simulink model "LiepkePlane"  (R2021a)
settings: Solver=FixedStepDiscrete  StartTime=0.0  StopTime=100  RelTol=1e-3  EnableMultiTasking=on
InitFcn:
  | runStart
StopFcn:
  | createGraphs
values from neighbouring files (symbols this model uses):
  alpha_matrix = data.alpha    [DatcomImport.m]
  alphai = trimAngle    (= -0.08927272)    [runStart.m]
  alt_matrix = data.alt    [DatcomImport.m]
  b = 8.0162    [runStart.m]
  beta = 0    [runStart.m]
  cbar = 4.3    [runStart.m]
  CD_0 = 0.0205    [runStart.m]
  CD_alpha = 0.058388    [runStart.m]
  CD_de = 0    [runStart.m]
  CD_ih = 0    [runStart.m]
  CD_q = 0    [runStart.m]
  CL_0 = 0.149    [runStart.m]
  Cl_0 = 0    [runStart.m]
  CL_alpha = 5.1265    [runStart.m]
  Cl_beta = -0.0301    [runStart.m]
  Cl_da = -0.1    [runStart.m]
  CL_de = 0.38    [runStart.m]
  Cl_dr = 0.05    [runStart.m]
  CL_ih = 0    [runStart.m]
  Cl_p = -0.5    [runStart.m]
  CL_q = 10.0    (= 10)    [runStart.m]
  Cl_r = 0.28    [runStart.m]
  cla_matrix = data.cla    [DatcomImport.m]
  clb_matrix = data.clb    [DatcomImport.m]
  clp_matrix = data.clp    [DatcomImport.m]
  clq_matrix = data.clq    [DatcomImport.m]
  clr_matrix = data.clr    [DatcomImport.m]
  Cm_0 = -0.08    [runStart.m]
  Cm_alpha = -0.3109    [runStart.m]
  Cm_de = -0.88    [runStart.m]
  Cm_ih = 0    [runStart.m]
  Cm_q = -17.7    [runStart.m]
  cma_matrix = data.cma    [DatcomImport.m]
  cmq_matrix = data.cmq    [DatcomImport.m]
  Cn_0 = 0    [runStart.m]
  Cn_beta = 0.1297    [runStart.m]
  Cn_da = 0.003    [runStart.m]
  Cn_dr = -0.18436    [runStart.m]
  Cn_p = - 0.09    (= -0.09)    [runStart.m]
  Cn_r = -0.26    [runStart.m]
  cnb_matrix = data.cnb    [DatcomImport.m]
  cnp_matrix = data.cnp    [DatcomImport.m]
  cnr_matrix = data.cnr    [DatcomImport.m]
  CY_0 = 0    [runStart.m]
  CY_beta = -.0301    (= -0.0301)    [runStart.m]
  CY_da = 0    [runStart.m]
  CY_dr = 0.0280    (= 0.028)    [runStart.m]
  CY_p = -0.140    (= -0.14)    [runStart.m]
  CY_r = 0.61    [runStart.m]
  cyb_matrix = data.cyb    [DatcomImport.m]
  cyp_matrix = data.cyp    [DatcomImport.m]
  H = 1981.2    [runStart.m]
  Ix = 1084.7    [runStart.m]
  Iy = 6507.9    [runStart.m]
  Iz = 7050.3    [runStart.m]
  Jxy = 0    [runStart.m]
  Jxz = 271.16    [runStart.m]
  Jyz = 0    [runStart.m]
  m = 2267.9    [runStart.m]
  mach_matrix = data.mach    [DatcomImport.m]
  p = 0    [runStart.m]
  phi = 0    [runStart.m]
  psi = 0    [runStart.m]
  q = 0    [runStart.m]
  r = 0    [runStart.m]
  S = 12.6348    [runStart.m]
  theta = trimAngle    (= -0.08927272)    [runStart.m]
  trimAngle = -8.927272e-02    (= -0.08927272)    [runStart.m]
  trimThrotte = 3.827652e-01    (= 0.3827652)    [runStart.m]
  v = 180    [runStart.m]
  xe = 0    [runStart.m]
  ye = 0    [runStart.m]
undefined symbols (not defined in the file or in its folder): DiscIntNeverNeededParam
libraries: airlib x2, aerolibfltsims x2, aerolibanimutils x2
(part 2 of 2)

== system LiepkePlane/ Liepke - AE 413 FInal/ae/aero/Stability 2 Body Axis ==
  alpha : Inport
  FsMb : Inport  Port=2
  Demux2 : Demux  Outputs=6
      settings: DisplayOption=none
  Mux1 : Mux  Inputs=6
  Product{2..5} (4 alike) : Product  InputSameDT=on  RndMeth=Zero  SaturateOnIntegerOverflow=on  OutDataTypeStr=Inherit: Same as first input
  Sum3 : Sum  Inputs=-+  InputSameDT=on  SaturateOnIntegerOverflow=on  OutDataTypeStr=Inherit: Same as first input
  Sum4 : Sum  Inputs=--  InputSameDT=on  SaturateOnIntegerOverflow=on  OutDataTypeStr=Inherit: Same as first input
  cos alpha : Fcn  Expr=cos(u[1])
  sin alpha : Fcn
  FbMb : Outport  VectorParamsAs1DForOutWhenUnconnected=off
  wires:
  Demux2/6 -> Mux1/6
  Demux2/5 -> Mux1/5
  Demux2/2 -> Mux1/2
  Demux2/4 -> Mux1/4
  cos alpha/1 -> Product2/1, Product5/1
  Demux2/1 -> Product2/2, Product4/2
  Product2/1 -> Sum3/1
  Product3/1 -> Sum3/2
  Sum3/1 -> Mux1/1
  sin alpha/1 -> Product3/1, Product4/1
  Demux2/3 -> Product3/2, Product5/2
  Product4/1 -> Sum4/1
  Product5/1 -> Sum4/2
  Sum4/1 -> Mux1/3
  alpha/1 -> sin alpha/1, cos alpha/1
  Mux1/1 -> FbMb/1
  FsMb/1 -> Demux2/1

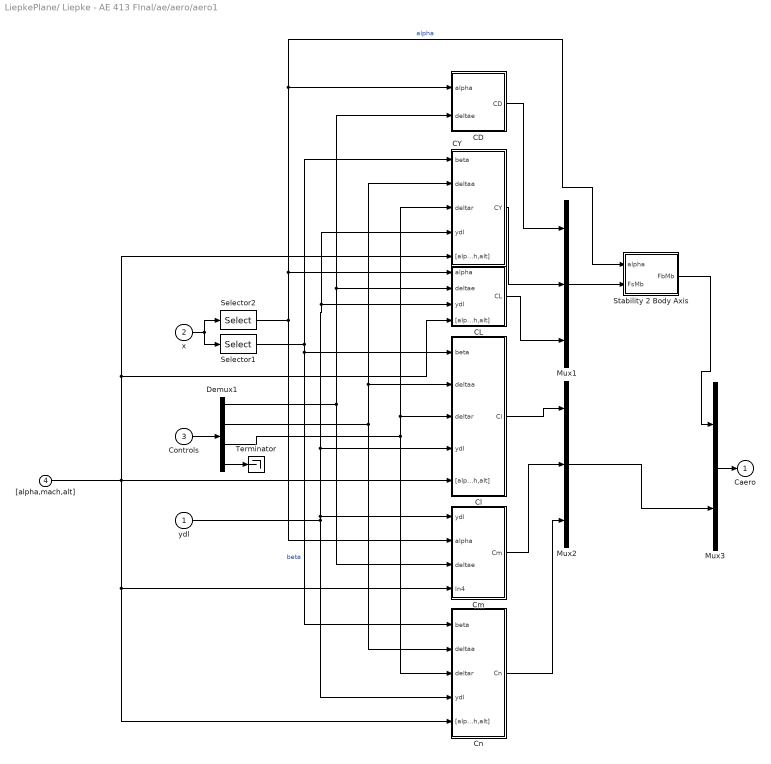
== system LiepkePlane/ Liepke - AE 413 FInal/ae/aero/aero1 ==
  ydl : Inport
  x : Inport  Port=2
  Controls : Inport  Port=3
  "[alpha,mach,alt]" : Inport  Port=4
  CD : Subsystem
  CL : Subsystem
  CY : Subsystem
  Cl : Subsystem
  Cm : Subsystem
  Cn : Subsystem
  Demux1 : Demux
      settings: DisplayOption=none
  Mux1 : Mux  Inputs=3
  Mux2 : Mux  Inputs=3
  Mux3 : Mux  Inputs=2
  Selector1 : Selector  InputPortWidth=12  IndexOptions=Index vector (dialog)  Indices=[3]  OutputSizes=1
  Selector2 : Selector  InputPortWidth=12  IndexOptions=Index vector (dialog)  Indices=[2]  OutputSizes=1
  Stability 2 Body Axis : Subsystem
  Terminator : Terminator
  Caero : Outport  VectorParamsAs1DForOutWhenUnconnected=off
  wires:
  Demux1/3 -> CY/3(deltar), Cl/3(deltar), Cn/3(deltar)
  Demux1/2 -> CY/2(deltaa), Cl/2(deltaa), Cn/2(deltaa)
  Demux1/1 -> CD/2(deltae), CL/2(deltae), Cm/3(deltae)
  ydl/1 -> CY/4(ydl), CL/3(ydl), Cl/4(ydl), Cm/1(ydl), Cn/4(ydl)
  CD/1(CD) -> Mux1/1
  Mux1/1 -> Stability 2 Body Axis/2(FsMb)
  CY/1(CY) -> Mux1/2
  x/1 -> Selector2/1, Selector1/1
  Selector1/1 -> Cn/1(beta), Cl/1(beta), CY/1(beta)  "beta"
  Selector2/1 -> Cm/2(alpha), Stability 2 Body Axis/1(alpha), CD/1(alpha), CL/1(alpha)  "alpha"
  CL/1(CL) -> Mux1/3
  Controls/1 -> Demux1/1
  Demux1/4 -> Terminator/1
  Stability 2 Body Axis/1(FbMb) -> Mux3/1
  Cl/1(Cl) -> Mux2/1
  Cm/1(Cm) -> Mux2/2
  Cn/1(Cn) -> Mux2/3
  Mux3/1 -> Caero/1
  Mux2/1 -> Mux3/2
  "[alpha,mach,alt]"/1 -> CY/5("[alpha,mach,alt]"), CL/4("[alpha,mach,alt]"), Cl/5("[alpha,mach,alt]"), Cn/5("[alpha,mach,alt]"), Cm/4(In4)

== system LiepkePlane/ Liepke - AE 413 FInal/ae/dl/0 ==

== system LiepkePlane/ Liepke - AE 413 FInal/ae/fmdims/0 ==

== system LiepkePlane/ Liepke - AE 413 FInal/eqm/ODE/0 ==

== system LiepkePlane/ Liepke - AE 413 FInal/eqm/ODE/Eulerdot ==
  note: ueul=[x;Ftot;Mtot;yhlp]
  note: yeul=[psi dot; theta dot; phi dot]
  ueul : Inport
  0 : Subsystem
      mask Display: disp('EULERDOT\nM.O. Rauw, October 1997')
  Mux1 : Mux  Inputs=[29 1]
  Mux2 : Mux  Inputs=3
  phi dot : Fcn  Expr=u[4] + u[30]*u[26]
  psi dot : Fcn  Expr=(u[5]*u[28] + u[6]*u[29])/u[27]
  theta dot : Fcn  Expr=u[5]*u[29] - u[6]*u[28]
  yeul : Outport
  wires:
  ueul/1 -> theta dot/1, Mux1/1, psi dot/1
  psi dot/1 -> Mux2/1, Mux1/2
  theta dot/1 -> Mux2/2
  Mux2/1 -> yeul/1
  phi dot/1 -> Mux2/3
  Mux1/1 -> phi dot/1

== system LiepkePlane/ Liepke - AE 413 FInal/eqm/ODE/Vabdot ==
  note: yVab=[V dot;alpha dot;beta dot]
  note: uVab=[x;Ftot;Mtot;yhlp]
  uVab : Inport
  0 : Subsystem
      mask Display: disp('VABDOT\nM.O. Rauw, October 1997')
  Mux2 : Mux  Inputs=3
  V dot : Fcn  Expr=(u[13]*u[19]*u[21]+u[14]*u[22]+u[15]*u[20]*u[21])/m
  alpha dot : Fcn  Expr=(-u[13]*u[20]+u[15]*u[19])/(m*u[1]*u[21]) - u[23]*(u[4]*u[19]+u[6]*u[20]) + u[5]
  beta dot : Fcn  Expr=(-u[13]*u[19]*u[22]+u[14]*u[21]-u[15]*u[20]*u[22])/(m*u[1]) + u[4]*u[20] - u[6]*u[19]
  yVab : Outport
  wires:
  beta dot/1 -> Mux2/3
  V dot/1 -> Mux2/1
  alpha dot/1 -> Mux2/2
  uVab/1 -> alpha dot/1, beta dot/1, V dot/1
  Mux2/1 -> yVab/1

== system LiepkePlane/ Liepke - AE 413 FInal/eqm/ODE/pqrdot ==
  note: ytmp = [L; M; N; p^2; pq; pr; q^2; qr; r^2]
  note: upqr=[x;Ftot;Mtot;yhlp]
  note: ypqr=[p dot;q dot;r dot]
  note: ytmp
  note: Here: ypqr = GM2*ytmp
  note: [L M N]'
  note: [p q r]'
  upqr : Inport
  0 : Subsystem
      mask Display: disp('PQRDOT\nM.O. Rauw, October 1997')
  Demux : Demux  Outputs=[3 3 9 3 11]
      settings: DisplayOption=none
  Fcn : Fcn  Expr=u[1]^2
  Fcn1 : Fcn  Expr=u[1]*u[2]
  Fcn2 : Fcn  Expr=u[1]*u[3]
  Fcn3 : Fcn  Expr=u[2]^2
  Fcn4 : Fcn  Expr=u[2]*u[3]
  Fcn5 : Fcn  Expr=u[3]^2
  "GM2 " : Subsystem  mask(State Space){M=GM2}
      mask prompts: M "Matrix"
      mask Display: disp('Matrix\nGain')
  Mux : Mux  Inputs=[3 1 1 1 1 1 1]
  Terminator1 : Terminator
  Terminator2 : Terminator
  Terminator3 : Terminator
  ypqr : Outport
  wires:
  Mux/1 -> "GM2 "/1(In1)
  "GM2 "/1(Out1) -> ypqr/1
  Fcn5/1 -> Mux/7
  Fcn4/1 -> Mux/6
  Fcn3/1 -> Mux/5
  Fcn2/1 -> Mux/4
  Fcn1/1 -> Mux/3
  Fcn/1 -> Mux/2
  Demux/4 -> Mux/1
  Demux/2 -> Fcn3/1, Fcn5/1, Fcn4/1, Fcn2/1, Fcn/1, Fcn1/1
  Demux/3 -> Terminator1/1
  Demux/5 -> Terminator2/1
  Demux/1 -> Terminator3/1
  upqr/1 -> Demux/1

== system LiepkePlane/ Liepke - AE 413 FInal/eqm/ODE/xyHdot ==
  note: uxyH=[x;Ftot;Mtot;yhlp]
  note: yxyH=[xe dot; ye dot; H dot]
  ybvel* : Inport
  uxYH : Inport  Port=2
  0 : Subsystem
      mask Display: disp('XYHDOT\nM.O. Rauw, October 1997')
  H dot : Fcn  Expr=u[30]*u[26] - (u[31]*u[28]+u[32]*u[29])*u[27]
  Mux2 : Mux  Inputs=[29 3]
  Mux3 : Mux  Inputs=2
  Mux4 : Mux  Inputs=[29 2]
  Mux5 : Mux  Inputs=3
  tmp1 : Fcn  Expr=u[30]*u[27] + (u[31]*u[28]+u[32]*u[29])*u[26]
  tmp2 : Fcn  Expr=u[31]*u[29] - u[32]*u[28]
  xe dot : Fcn  Expr=u[30]*u[25] - u[31]*u[24]
  ye dot : Fcn  Expr=u[30]*u[24] + u[31]*u[25]
  yxyH : Outport
  wires:
  uxYH/1 -> Mux2/1, Mux4/1
  ybvel*/1 -> Mux2/2
  Mux3/1 -> Mux4/2
  Mux2/1 -> tmp1/1, tmp2/1, H dot/1
  Mux4/1 -> xe dot/1, ye dot/1
  Mux5/1 -> yxyH/1
  ye dot/1 -> Mux5/2
  tmp2/1 -> Mux3/2
  xe dot/1 -> Mux5/1
  H dot/1 -> Mux5/3
  tmp1/1 -> Mux3/1

== system LiepkePlane/ Liepke - AE 413 FInal/eqm/uvw/0 ==

== system LiepkePlane/ Liepke - AE 413 FInal/eqm/xdotcorr/0 ==

== system LiepkePlane/ Liepke - AE 413 FInal/out/accel/0 ==

== system LiepkePlane/ Liepke - AE 413 FInal/out/fp/0 ==

== system LiepkePlane/ Liepke - AE 413 FInal/out/uvwdot/0 ==

== system LiepkePlane/ Liepke - AE 413 FInal/ae/aero/aero1/CD ==
  alpha : Inport
  deltae : Inport  Port=2
  CLa : Constant  Value=CD_alpha  SampleTime=-1
  CLa1 : Constant  Value=CD_0  SampleTime=-1
  CLde : Constant  Value=CD_de  SampleTime=-1
  Sum2 : Sum  Inputs=+++  InputSameDT=on  SaturateOnIntegerOverflow=on  OutDataTypeStr=Inherit: Same as first input
  n : Product  InputSameDT=on  SaturateOnIntegerOverflow=on  OutDataTypeStr=Inherit: Same as first input
  n1 : Product  InputSameDT=on  SaturateOnIntegerOverflow=on  OutDataTypeStr=Inherit: Same as first input
  CD : Outport  VectorParamsAs1DForOutWhenUnconnected=off
  wires:
  n/1 -> Sum2/2
  Sum2/1 -> CD/1
  n1/1 -> Sum2/1
  CLa1/1 -> Sum2/3
  alpha/1 -> n/1
  CLa/1 -> n/2
  deltae/1 -> n1/1
  CLde/1 -> n1/2

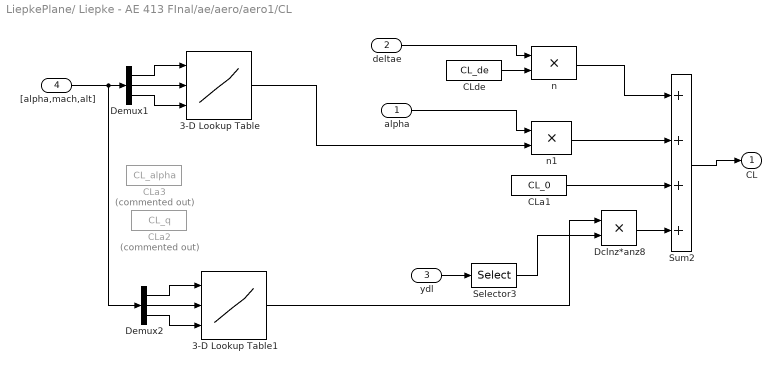
== system LiepkePlane/ Liepke - AE 413 FInal/ae/aero/aero1/CL ==
  alpha : Inport
  deltae : Inport  Port=2
  ydl : Inport  Port=3
  "[alpha,mach,alt]" : Inport  Port=4
  3-D Lookup Table : Lookup_n-D  NumberOfTableDimensions=3  BreakpointsForDimension1=alpha_matrix  BreakpointsForDimension2=mach_matrix  BreakpointsForDimension3=alt_matrix  Table=cla_matrix  InternalRulePriority=Speed  RndMeth=Simplest  InputSameDT=on
      settings: InputPortMap=u0,u1,u2
  3-D Lookup Table1 : Lookup_n-D  NumberOfTableDimensions=3  BreakpointsForDimension1=alpha_matrix  BreakpointsForDimension2=mach_matrix  BreakpointsForDimension3=alt_matrix  Table=clq_matrix  InternalRulePriority=Speed  RndMeth=Simplest  InputSameDT=on
      settings: InputPortMap=u0,u1,u2
  CLa1 : Constant  Value=CL_0  SampleTime=-1
  CLa2 : Constant  Commented=on  Value=CL_q  SampleTime=-1
  CLa3 : Constant  Commented=on  Value=CL_alpha  SampleTime=-1
  CLde : Constant  Value=CL_de  SampleTime=-1
  Dclnz*anz8 : Product  InputSameDT=on  SaturateOnIntegerOverflow=on  OutDataTypeStr=Inherit: Same as first input
  Demux1 : Demux  Outputs=3
  Demux2 : Demux  Outputs=3
  Selector3 : Selector  InputPortWidth=3  IndexOptions=Index vector (dialog)  Indices=[2]  OutputSizes=1
  Sum2 : Sum  Inputs=++++  InputSameDT=on  SaturateOnIntegerOverflow=on  OutDataTypeStr=Inherit: Same as first input
  n : Product  InputSameDT=on  SaturateOnIntegerOverflow=on  OutDataTypeStr=Inherit: Same as first input
  n1 : Product  InputSameDT=on  SaturateOnIntegerOverflow=on  OutDataTypeStr=Inherit: Same as first input
  CL : Outport  VectorParamsAs1DForOutWhenUnconnected=off
  wires:
  CLa1/1 -> Sum2/3
  n/1 -> Sum2/1
  Sum2/1 -> CL/1
  n1/1 -> Sum2/2
  Dclnz*anz8/1 -> Sum2/4
  Selector3/1 -> Dclnz*anz8/2
  ydl/1 -> Selector3/1
  deltae/1 -> n/1
  CLde/1 -> n/2
  alpha/1 -> n1/1
  Demux1/1 -> 3-D Lookup Table/1
  Demux1/3 -> 3-D Lookup Table/3
  Demux1/2 -> 3-D Lookup Table/2
  "[alpha,mach,alt]"/1 -> Demux2/1, Demux1/1
  3-D Lookup Table/1 -> n1/2
  Demux2/2 -> 3-D Lookup Table1/2
  Demux2/3 -> 3-D Lookup Table1/3
  Demux2/1 -> 3-D Lookup Table1/1
  3-D Lookup Table1/1 -> Dclnz*anz8/1

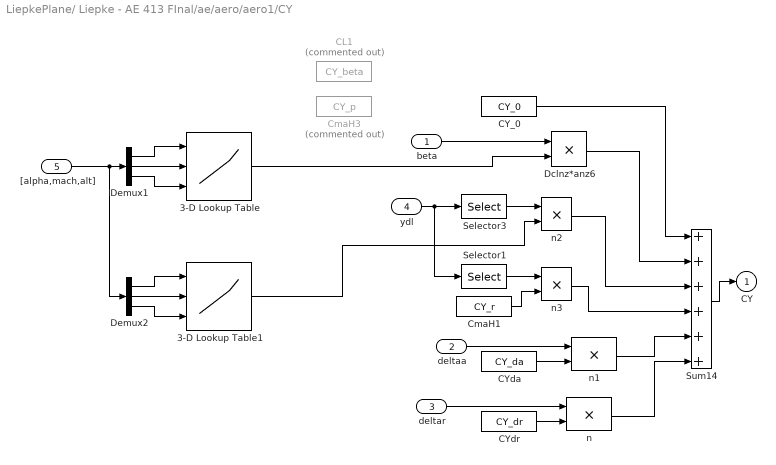
== system LiepkePlane/ Liepke - AE 413 FInal/ae/aero/aero1/CY ==
  beta : Inport
  deltaa : Inport  Port=2
  deltar : Inport  Port=3
  ydl : Inport  Port=4
  "[alpha,mach,alt]" : Inport  Port=5
  3-D Lookup Table : Lookup_n-D  NumberOfTableDimensions=3  BreakpointsForDimension1=alpha_matrix  BreakpointsForDimension2=mach_matrix  BreakpointsForDimension3=alt_matrix  Table=cyb_matrix  InternalRulePriority=Speed  RndMeth=Simplest  InputSameDT=on
      settings: InputPortMap=u0,u1,u2
  3-D Lookup Table1 : Lookup_n-D  NumberOfTableDimensions=3  BreakpointsForDimension1=alpha_matrix  BreakpointsForDimension2=mach_matrix  BreakpointsForDimension3=alt_matrix  Table=cyp_matrix  InternalRulePriority=Speed  RndMeth=Simplest  InputSameDT=on
      settings: InputPortMap=u0,u1,u2
  CL1 : Constant  Commented=on  Value=CY_beta
  CY_0 : Constant  Value=CY_0
  CYda : Constant  Value=CY_da
  CYdr : Constant  Value=CY_dr
  CmaH1 : Constant  Value=CY_r
  CmaH3 : Constant  Commented=on  Value=CY_p
  Dclnz*anz6 : Product  InputSameDT=on  SaturateOnIntegerOverflow=on  OutDataTypeStr=Inherit: Same as first input
  Demux1 : Demux  Outputs=3
  Demux2 : Demux  Outputs=3
  Selector1 : Selector  InputPortWidth=3  IndexOptions=Index vector (dialog)  Indices=3  OutputSizes=1
  Selector3 : Selector  InputPortWidth=3  IndexOptions=Index vector (dialog)  Indices=1  OutputSizes=1
  Sum14 : Sum  Inputs=6  InputSameDT=on  SaturateOnIntegerOverflow=on  OutDataTypeStr=Inherit: Same as first input
  n{,1..3} (4 alike) : Product  InputSameDT=on  SaturateOnIntegerOverflow=on  OutDataTypeStr=Inherit: Same as first input
  CY : Outport  VectorParamsAs1DForOutWhenUnconnected=off
  wires:
  beta/1 -> Dclnz*anz6/1
  CYdr/1 -> n/2
  deltar/1 -> n/1
  CYda/1 -> n1/2
  deltaa/1 -> n1/1
  3-D Lookup Table1/1 -> n2/2
  Selector3/1 -> n2/1
  ydl/1 -> Selector1/1, Selector3/1
  Selector1/1 -> n3/1
  CmaH1/1 -> n3/2
  Sum14/1 -> CY/1
  Dclnz*anz6/1 -> Sum14/2
  CY_0/1 -> Sum14/1
  n2/1 -> Sum14/3
  n3/1 -> Sum14/4
  n1/1 -> Sum14/5
  n/1 -> Sum14/6
  Demux1/1 -> 3-D Lookup Table/1
  Demux1/3 -> 3-D Lookup Table/3
  "[alpha,mach,alt]"/1 -> Demux2/1, Demux1/1
  Demux1/2 -> 3-D Lookup Table/2
  3-D Lookup Table/1 -> Dclnz*anz6/2
  Demux2/3 -> 3-D Lookup Table1/3
  Demux2/2 -> 3-D Lookup Table1/2
  Demux2/1 -> 3-D Lookup Table1/1

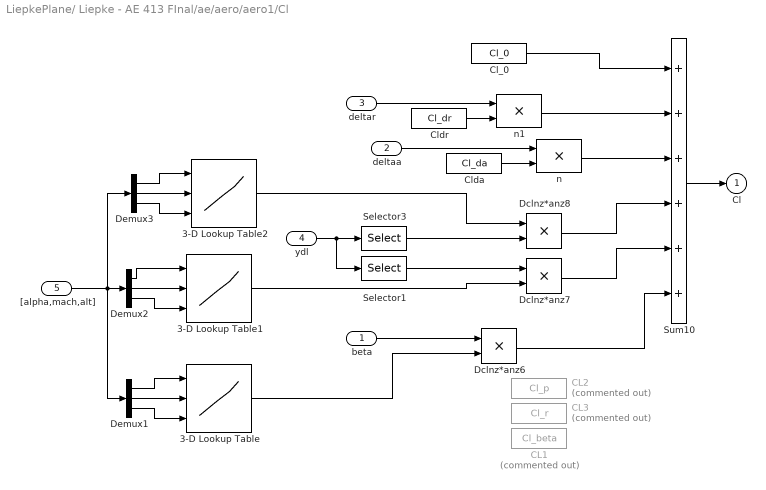
== system LiepkePlane/ Liepke - AE 413 FInal/ae/aero/aero1/Cl ==
  beta : Inport
  deltaa : Inport  Port=2
  deltar : Inport  Port=3
  ydl : Inport  Port=4
  "[alpha,mach,alt]" : Inport  Port=5
  3-D Lookup Table : Lookup_n-D  NumberOfTableDimensions=3  BreakpointsForDimension1=alpha_matrix  BreakpointsForDimension2=mach_matrix  BreakpointsForDimension3=alt_matrix  Table=clb_matrix  InternalRulePriority=Speed  RndMeth=Simplest  InputSameDT=on
      settings: InputPortMap=u0,u1,u2
  3-D Lookup Table1 : Lookup_n-D  NumberOfTableDimensions=3  BreakpointsForDimension1=alpha_matrix  BreakpointsForDimension2=mach_matrix  BreakpointsForDimension3=alt_matrix  Table=clr_matrix  InternalRulePriority=Speed  RndMeth=Simplest  InputSameDT=on
      settings: InputPortMap=u0,u1,u2
  3-D Lookup Table2 : Lookup_n-D  NumberOfTableDimensions=3  BreakpointsForDimension1=alpha_matrix  BreakpointsForDimension2=mach_matrix  BreakpointsForDimension3=alt_matrix  Table=clp_matrix  InternalRulePriority=Speed  RndMeth=Simplest  InputSameDT=on
      settings: InputPortMap=u0,u1,u2
  CL1 : Constant  Commented=on  Value=Cl_beta
  CL2 : Constant  Commented=on  Value=Cl_p
  CL3 : Constant  Commented=on  Value=Cl_r
  Cl_0 : Constant  Value=Cl_0
  Clda : Constant  Value=Cl_da
  Cldr : Constant  Value=Cl_dr
  Dclnz*anz6 : Product  InputSameDT=on  SaturateOnIntegerOverflow=on  OutDataTypeStr=Inherit: Same as first input
  Dclnz*anz7 : Product  InputSameDT=on  SaturateOnIntegerOverflow=on  OutDataTypeStr=Inherit: Same as first input
  Dclnz*anz8 : Product  InputSameDT=on  SaturateOnIntegerOverflow=on  OutDataTypeStr=Inherit: Same as first input
  Demux1 : Demux  Outputs=3
  Demux2 : Demux  Outputs=3
  Demux3 : Demux  Outputs=3
  Selector1 : Selector  InputPortWidth=3  IndexOptions=Index vector (dialog)  Indices=[3]  OutputSizes=1
  Selector3 : Selector  InputPortWidth=3  IndexOptions=Index vector (dialog)  Indices=[1]  OutputSizes=1
  Sum10 : Sum  Inputs=++++++  InputSameDT=on  SaturateOnIntegerOverflow=on  OutDataTypeStr=Inherit: Same as first input
  n : Product  InputSameDT=on  SaturateOnIntegerOverflow=on  OutDataTypeStr=Inherit: Same as first input
  n1 : Product  InputSameDT=on  SaturateOnIntegerOverflow=on  OutDataTypeStr=Inherit: Same as first input
  Cl : Outport  VectorParamsAs1DForOutWhenUnconnected=off
  wires:
  n/1 -> Sum10/3
  Dclnz*anz7/1 -> Sum10/5
  Dclnz*anz8/1 -> Sum10/4
  Sum10/1 -> Cl/1
  Dclnz*anz6/1 -> Sum10/6
  ydl/1 -> Selector1/1, Selector3/1
  3-D Lookup Table1/1 -> Dclnz*anz7/2
  Selector1/1 -> Dclnz*anz7/1
  Selector3/1 -> Dclnz*anz8/2
  n1/1 -> Sum10/2
  beta/1 -> Dclnz*anz6/1
  deltaa/1 -> n/1
  Clda/1 -> n/2
  Cldr/1 -> n1/2
  deltar/1 -> n1/1
  Cl_0/1 -> Sum10/1
  Demux1/1 -> 3-D Lookup Table/1
  Demux1/3 -> 3-D Lookup Table/3
  Demux1/2 -> 3-D Lookup Table/2
  "[alpha,mach,alt]"/1 -> Demux2/1, Demux1/1, Demux3/1
  3-D Lookup Table/1 -> Dclnz*anz6/2
  Demux2/3 -> 3-D Lookup Table1/3
  Demux2/2 -> 3-D Lookup Table1/2
  Demux2/1 -> 3-D Lookup Table1/1
  Demux3/3 -> 3-D Lookup Table2/3
  Demux3/2 -> 3-D Lookup Table2/2
  Demux3/1 -> 3-D Lookup Table2/1
  3-D Lookup Table2/1 -> Dclnz*anz8/1

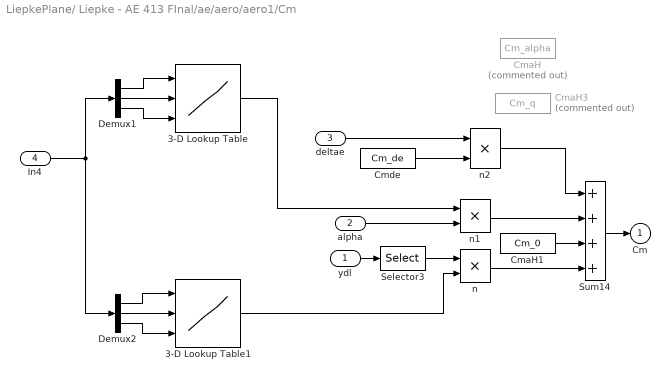
== system LiepkePlane/ Liepke - AE 413 FInal/ae/aero/aero1/Cm ==
  ydl : Inport
  alpha : Inport  Port=2
  deltae : Inport  Port=3
  In4 : Inport  Port=4
  3-D Lookup Table : Lookup_n-D  NumberOfTableDimensions=3  BreakpointsForDimension1=alpha_matrix  BreakpointsForDimension2=mach_matrix  BreakpointsForDimension3=alt_matrix  Table=cma_matrix  InternalRulePriority=Speed  RndMeth=Simplest  InputSameDT=on
      settings: InputPortMap=u0,u1,u2
  3-D Lookup Table1 : Lookup_n-D  NumberOfTableDimensions=3  BreakpointsForDimension1=alpha_matrix  BreakpointsForDimension2=mach_matrix  BreakpointsForDimension3=alt_matrix  Table=cmq_matrix  InternalRulePriority=Speed  RndMeth=Simplest  InputSameDT=on
      settings: InputPortMap=u0,u1,u2
  CmaH : Constant  Commented=on  Value=Cm_alpha
  CmaH1 : Constant  Value=Cm_0
  CmaH3 : Constant  Commented=on  Value=Cm_q
  Cmde : Constant  Value=Cm_de
  Demux1 : Demux  Outputs=3
  Demux2 : Demux  Outputs=3
  Selector3 : Selector  InputPortWidth=3  IndexOptions=Index vector (dialog)  Indices=[2]  OutputSizes=1
  Sum14 : Sum  Inputs=++++  InputSameDT=on  SaturateOnIntegerOverflow=on  OutDataTypeStr=Inherit: Same as first input
  n : Product  InputSameDT=on  SaturateOnIntegerOverflow=on  OutDataTypeStr=Inherit: Same as first input
  n1 : Product  InputSameDT=on  SaturateOnIntegerOverflow=on  OutDataTypeStr=Inherit: Same as first input
  n2 : Product  InputSameDT=on  SaturateOnIntegerOverflow=on  OutDataTypeStr=Inherit: Same as first input
  Cm : Outport  VectorParamsAs1DForOutWhenUnconnected=off
  wires:
  Selector3/1 -> n/1
  n1/1 -> Sum14/2
  ydl/1 -> Selector3/1
  n/1 -> Sum14/4
  Sum14/1 -> Cm/1
  CmaH1/1 -> Sum14/3
  alpha/1 -> n1/2
  Cmde/1 -> n2/2
  n2/1 -> Sum14/1
  deltae/1 -> n2/1
  Demux1/2 -> 3-D Lookup Table/2
  Demux1/3 -> 3-D Lookup Table/3
  Demux1/1 -> 3-D Lookup Table/1
  Demux2/1 -> 3-D Lookup Table1/1
  Demux2/3 -> 3-D Lookup Table1/3
  Demux2/2 -> 3-D Lookup Table1/2
  In4/1 -> Demux1/1, Demux2/1
  3-D Lookup Table1/1 -> n/2
  3-D Lookup Table/1 -> n1/1

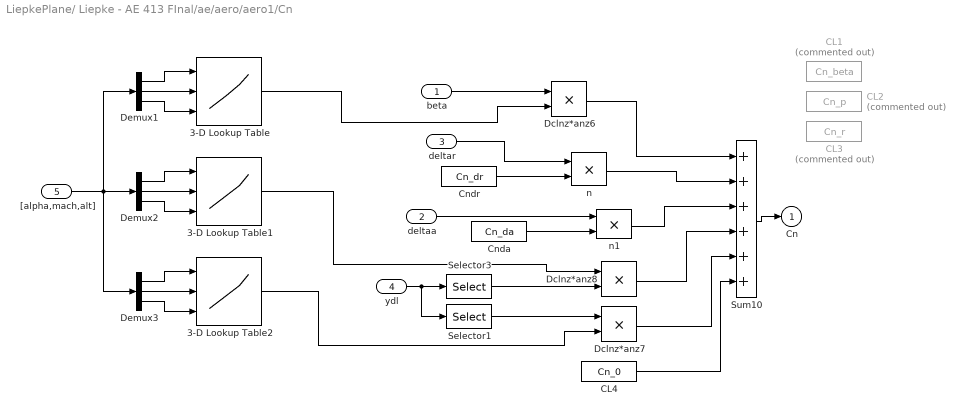
== system LiepkePlane/ Liepke - AE 413 FInal/ae/aero/aero1/Cn ==
  beta : Inport
  deltaa : Inport  Port=2
  deltar : Inport  Port=3
  ydl : Inport  Port=4
  "[alpha,mach,alt]" : Inport  Port=5
  3-D Lookup Table : Lookup_n-D  NumberOfTableDimensions=3  BreakpointsForDimension1=alpha_matrix  BreakpointsForDimension2=mach_matrix  BreakpointsForDimension3=alt_matrix  Table=cnb_matrix  InternalRulePriority=Speed  RndMeth=Simplest  InputSameDT=on
      settings: InputPortMap=u0,u1,u2
  3-D Lookup Table1 : Lookup_n-D  NumberOfTableDimensions=3  BreakpointsForDimension1=alpha_matrix  BreakpointsForDimension2=mach_matrix  BreakpointsForDimension3=alt_matrix  Table=cnp_matrix  InternalRulePriority=Speed  RndMeth=Simplest  InputSameDT=on
      settings: InputPortMap=u0,u1,u2
  3-D Lookup Table2 : Lookup_n-D  NumberOfTableDimensions=3  BreakpointsForDimension1=alpha_matrix  BreakpointsForDimension2=mach_matrix  BreakpointsForDimension3=alt_matrix  Table=cnr_matrix  InternalRulePriority=Speed  RndMeth=Simplest  InputSameDT=on
      settings: InputPortMap=u0,u1,u2
  CL1 : Constant  Commented=on  Value=Cn_beta  SampleTime=-1
  CL2 : Constant  Commented=on  Value=Cn_p
  CL3 : Constant  Commented=on  Value=Cn_r
  CL4 : Constant  Value=Cn_0  SampleTime=-1
  Cnda : Constant  Value=Cn_da  SampleTime=-1
  Cndr : Constant  Value=Cn_dr  SampleTime=-1
  Dclnz*anz6 : Product  InputSameDT=on  SaturateOnIntegerOverflow=on  OutDataTypeStr=Inherit: Same as first input
  Dclnz*anz7 : Product  InputSameDT=on  SaturateOnIntegerOverflow=on  OutDataTypeStr=Inherit: Same as first input
  Dclnz*anz8 : Product  InputSameDT=on  SaturateOnIntegerOverflow=on  OutDataTypeStr=Inherit: Same as first input
  Demux1 : Demux  Outputs=3
  Demux2 : Demux  Outputs=3
  Demux3 : Demux  Outputs=3
  Selector1 : Selector  InputPortWidth=3  IndexOptions=Index vector (dialog)  Indices=[3]  OutputSizes=1
  Selector3 : Selector  InputPortWidth=3  IndexOptions=Index vector (dialog)  Indices=[1]  OutputSizes=1
  Sum10 : Sum  Inputs=6  InputSameDT=on  SaturateOnIntegerOverflow=on  OutDataTypeStr=Inherit: Same as first input
  n : Product  InputSameDT=on  SaturateOnIntegerOverflow=on  OutDataTypeStr=Inherit: Same as first input
  n1 : Product  InputSameDT=on  SaturateOnIntegerOverflow=on  OutDataTypeStr=Inherit: Same as first input
  Cn : Outport  VectorParamsAs1DForOutWhenUnconnected=off
  wires:
  beta/1 -> Dclnz*anz6/1
  Selector3/1 -> Dclnz*anz8/2
  Selector1/1 -> Dclnz*anz7/1
  ydl/1 -> Selector3/1, Selector1/1
  Dclnz*anz6/1 -> Sum10/1
  Sum10/1 -> Cn/1
  Dclnz*anz8/1 -> Sum10/4
  Dclnz*anz7/1 -> Sum10/5
  n1/1 -> Sum10/3
  deltar/1 -> n/1
  Cndr/1 -> n/2
  n/1 -> Sum10/2
  Cnda/1 -> n1/2
  deltaa/1 -> n1/1
  CL4/1 -> Sum10/6
  Demux1/1 -> 3-D Lookup Table/1
  Demux1/3 -> 3-D Lookup Table/3
  Demux1/2 -> 3-D Lookup Table/2
  "[alpha,mach,alt]"/1 -> Demux3/1, Demux2/1, Demux1/1
  3-D Lookup Table/1 -> Dclnz*anz6/2
  Demux2/3 -> 3-D Lookup Table1/3
  Demux2/1 -> 3-D Lookup Table1/1
  Demux2/2 -> 3-D Lookup Table1/2
  Demux3/3 -> 3-D Lookup Table2/3
  Demux3/1 -> 3-D Lookup Table2/1
  Demux3/2 -> 3-D Lookup Table2/2
  3-D Lookup Table2/1 -> Dclnz*anz7/2
  3-D Lookup Table1/1 -> Dclnz*anz8/1

== system LiepkePlane/ Liepke - AE 413 FInal/ae/aero/aero1/Stability 2 Body Axis ==
  alpha : Inport
  FsMb : Inport  Port=2
  Demux2 : Demux  Outputs=3
      settings: DisplayOption=none
  Mux1 : Mux  Inputs=3
  Product{2..5} (4 alike) : Product  InputSameDT=on  RndMeth=Zero  SaturateOnIntegerOverflow=on  OutDataTypeStr=Inherit: Same as first input
  Sum3 : Sum  Inputs=-+  InputSameDT=on  SaturateOnIntegerOverflow=on  OutDataTypeStr=Inherit: Same as first input
  Sum4 : Sum  Inputs=--  InputSameDT=on  SaturateOnIntegerOverflow=on  OutDataTypeStr=Inherit: Same as first input
  cos alpha : Fcn  Expr=cos(u[1])
  sin alpha : Fcn
  FbMb : Outport  VectorParamsAs1DForOutWhenUnconnected=off
  wires:
  Demux2/2 -> Mux1/2
  cos alpha/1 -> Product2/1, Product5/1
  Demux2/1 -> Product2/2, Product4/2
  Product2/1 -> Sum3/1
  Product3/1 -> Sum3/2
  Sum3/1 -> Mux1/1
  sin alpha/1 -> Product3/1, Product4/1
  Demux2/3 -> Product3/2, Product5/2
  Product4/1 -> Sum4/1
  Product5/1 -> Sum4/2
  Sum4/1 -> Mux1/3
  alpha/1 -> sin alpha/1, cos alpha/1
  Mux1/1 -> FbMb/1
  FsMb/1 -> Demux2/1

== system LiepkePlane/ Liepke - AE 413 FInal/eqm/ODE/Eulerdot/0 ==

== system LiepkePlane/ Liepke - AE 413 FInal/eqm/ODE/Vabdot/0 ==

== system LiepkePlane/ Liepke - AE 413 FInal/eqm/ODE/pqrdot/0 ==

== system LiepkePlane/ Liepke - AE 413 FInal/eqm/ODE/pqrdot/GM2  ==
  In1 : Inport
  Matrix Gain : StateSpace  A=[]  B=[]  C=[]  D=M  InitialCondition=0
  Out1 : Outport
  wires:
  In1/1 -> Matrix Gain/1
  Matrix Gain/1 -> Out1/1

== system LiepkePlane/ Liepke - AE 413 FInal/eqm/ODE/xyHdot/0 ==
